simulink subsystem "HDS_DrawCrosshair"  (R2019b)
settings: Solver=VariableStepAuto  StartTime=0.0  StopTime=10.0  RelTol=1e-3
settings Model: Creator=toons  LastModifiedBy=toons

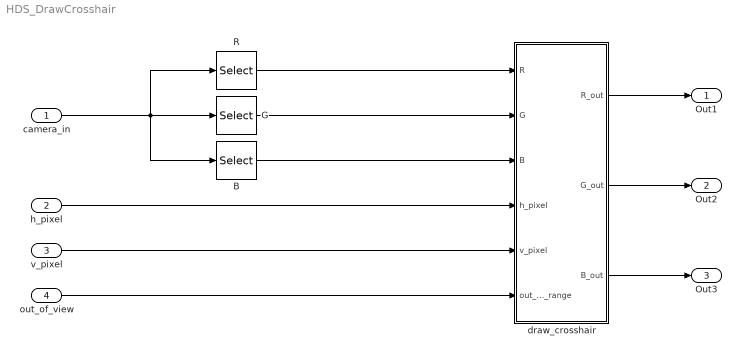
== system HDS_DrawCrosshair ==
  camera_in : Inport
  h_pixel : Inport  Port=2
  v_pixel : Inport  Port=3
  out_of_view : Inport  Port=4
  B : Selector  NumberOfDimensions=3  InputPortWidth=3  IndexOptions=Select all,Select all,Index vector (dialog)  Indices=[1 3],1,3  OutputSizes=1,1,1
  G : Selector  NumberOfDimensions=3  InputPortWidth=3  IndexOptions=Select all,Select all,Index vector (dialog)  Indices=[1 3],1,2  OutputSizes=1,1,1
  R : Selector  NumberOfDimensions=3  InputPortWidth=3  IndexOptions=Select all,Select all,Index vector (dialog)  Indices=[1 3],1,1  OutputSizes=1,1,1
  draw_crosshair : Subsystem
  Out1 : Outport
  Out2 : Outport  Port=2
  Out3 : Outport  Port=3
  wires:
  camera_in/1 -> R/1, G/1, B/1
  R/1 -> draw_crosshair/1(R)
  G/1 -> draw_crosshair/2(G)
  B/1 -> draw_crosshair/3(B)
  h_pixel/1 -> draw_crosshair/4(h_pixel)
  v_pixel/1 -> draw_crosshair/5(v_pixel)
  out_of_view/1 -> draw_crosshair/6(out_of_range)
  draw_crosshair/1(R_out) -> Out1/1
  draw_crosshair/2(G_out) -> Out2/1
  draw_crosshair/3(B_out) -> Out3/1

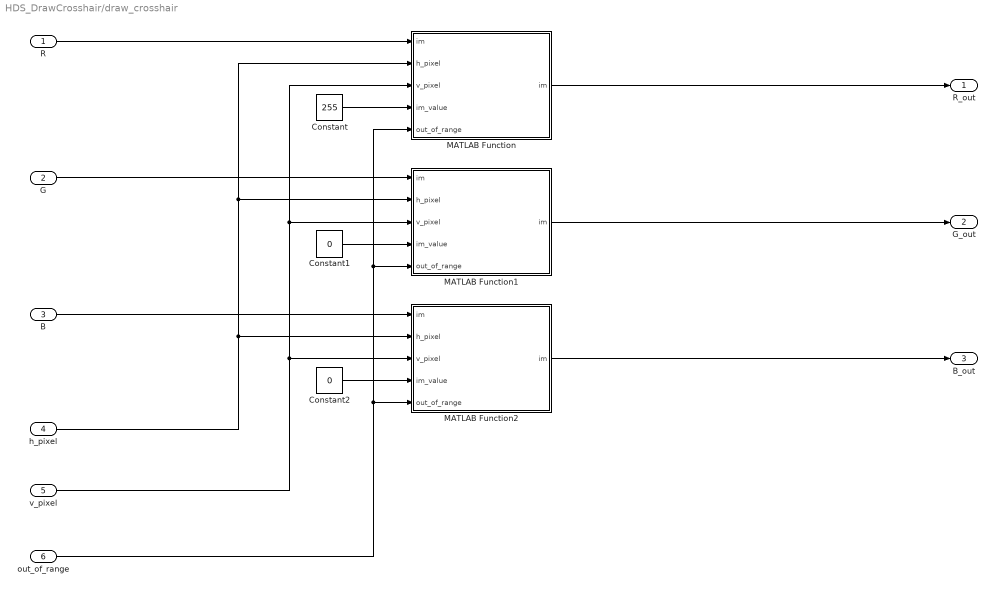
== system HDS_DrawCrosshair/draw_crosshair ==
  R : Inport
  G : Inport  Port=2
  B : Inport  Port=3
  h_pixel : Inport  Port=4
  v_pixel : Inport  Port=5
  out_of_range : Inport  Port=6
  Constant : Constant  Value=255
  Constant1 : Constant  Value=0
  Constant2 : Constant  Value=0
  MATLAB Function : MATLAB Function  TreatAsAtomicUnit=on
  MATLAB Function1 : MATLAB Function  TreatAsAtomicUnit=on
  MATLAB Function2 : MATLAB Function  TreatAsAtomicUnit=on
  R_out : Outport
  G_out : Outport  Port=2
  B_out : Outport  Port=3
  wires:
  R/1 -> MATLAB Function/1("im ")
  h_pixel/1 -> MATLAB Function2/2(h_pixel), MATLAB Function/2(h_pixel), MATLAB Function1/2(h_pixel)
  v_pixel/1 -> MATLAB Function2/3(v_pixel), MATLAB Function1/3(v_pixel), MATLAB Function/3(v_pixel)
  out_of_range/1 -> MATLAB Function2/5(out_of_range), MATLAB Function1/5(out_of_range), MATLAB Function/5(out_of_range)
  Constant/1 -> MATLAB Function/4(im_value)
  MATLAB Function/1(im) -> R_out/1
  G/1 -> MATLAB Function1/1("im ")
  B/1 -> MATLAB Function2/1("im ")
  Constant1/1 -> MATLAB Function1/4(im_value)
  Constant2/1 -> MATLAB Function2/4(im_value)
  MATLAB Function2/1(im) -> B_out/1
  MATLAB Function1/1(im) -> G_out/1

== matlab function HDS_DrawCrosshair/draw_crosshair/MATLAB Function ==
  data: im input; im output; h_pixel input; v_pixel input; im_value input; out_of_range input
function im = draw_crosshair(im, h_pixel, v_pixel, im_value, out_of_range)

if out_of_range == 0
    im(:,h_pixel) = im_value;
    im(v_pixel,:) = im_value;
end

== matlab function HDS_DrawCrosshair/draw_crosshair/MATLAB Function1 ==
  data: im input; im output; h_pixel input; v_pixel input; im_value input; out_of_range input
function im = draw_crosshair(im, h_pixel, v_pixel, im_value, out_of_range)

if out_of_range == 0
    im(:,h_pixel) = im_value;
    im(v_pixel,:) = im_value;
end

== matlab function HDS_DrawCrosshair/draw_crosshair/MATLAB Function2 ==
  data: im input; im output; h_pixel input; v_pixel input; im_value input; out_of_range input
function im = draw_crosshair(im, h_pixel, v_pixel, im_value, out_of_range)

if out_of_range == 0
    im(:,h_pixel) = im_value;
    im(v_pixel,:) = im_value;
end
